simulink model "positive_negative_step_counters"  (R2019a)
settings: Solver=FixedStepDiscrete  StartTime=0.0  StopTime=50  FixedStep=1  RelTol=1e-3
settings Model: Creator=Suhas  LastModifiedBy=Suhas

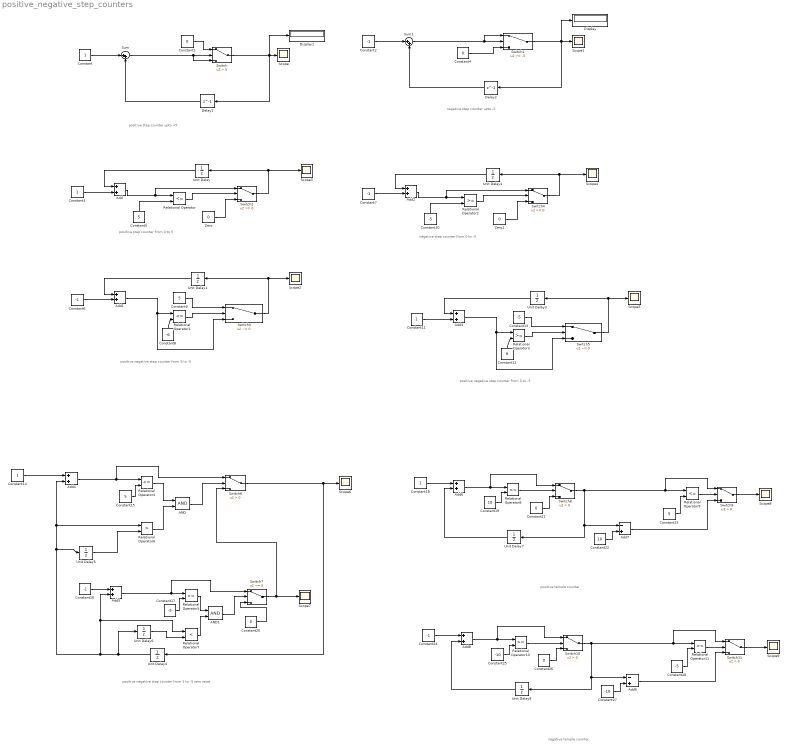
== system positive_negative_step_counters ==
  note: positive temple counter
  note: positive step counter from 0 to 5
  note: positive step counter upto +5
  note: negative step counter upto -5
  note: negative step counter from 0 to -5
  note: positive negative step counter from 5 to -5
  note: positive negative step counter from 5 to -5
  note: positive negative step counter from 5 to -5 zero reset
  note: negative temple counter
  AND : Logic  AllPortsSameDT=off  OutDataTypeStr=boolean
  AND1 : Logic  AllPortsSameDT=off  OutDataTypeStr=boolean
  Add{,1..6,8} (8 alike) : Sum
  Add7 : Sum  Inputs=-+
  Add9 : Sum  Inputs=-+
  Constant{,3,11,14,18} (5 alike) : Constant
  Constant{1,4,20..21,26} (5 alike) : Constant  Value=0
  Constant{10,13,17,28} (4 alike) : Constant  Value=-5
  Constant12 : Constant  Value=6
  Constant{5,9,15,23} (4 alike) : Constant  Value=5
  Constant{2,6..7,16,24} (5 alike) : Constant  Value=-1
  Constant19 : Constant  Value=10
  Constant22 : Constant  Value=10
  Constant25 : Constant  Value=-10
  Constant27 : Constant  Value=-10
  Constant8 : Constant  Value=-6
  Delay1 : Delay  DelayLength=1  InitialCondition=-1
  Delay2 : Delay  DelayLength=1  InitialCondition=1
  Display : Display
  Display1 : Display
  Relational Operator{,1,4,8..9} (5 alike) : RelationalOperator  Operator=<=  OutDataTypeStr=boolean  RndMeth=Simplest
  Relational Operator{2..3,5,10..11} (5 alike) : RelationalOperator  OutDataTypeStr=boolean  RndMeth=Simplest
  Relational Operator6 : RelationalOperator  Operator=>  OutDataTypeStr=boolean  RndMeth=Simplest
  Relational Operator7 : RelationalOperator  Operator=<  OutDataTypeStr=boolean  RndMeth=Simplest
  Scope{,1..9} (10 alike) : Scope
  Sum : Sum  Inputs=|++
  Sum1 : Sum  Inputs=|++
  Switch : Switch  Criteria=u2 > Threshold  Threshold=5
  Switch1 : Switch  Threshold=-5
  Switch{6,8..11} (5 alike) : Switch  Criteria=u2 > Threshold
  Switch2 : Switch
  Switch3 : Switch  Criteria=u2 ~= 0
  Switch4 : Switch
  Switch5 : Switch  Criteria=u2 ~= 0
  Switch7 : Switch  Criteria=u2 ~= 0
  Unit Delay{,3..4,7} (4 alike) : UnitDelay  InitialCondition=-1  SampleTime=-1  HasFrameUpgradeWarning=on
  Unit Delay1 : UnitDelay  InitialCondition=1  SampleTime=-1  HasFrameUpgradeWarning=on
  Unit Delay2 : UnitDelay  InitialCondition=1  SampleTime=-1  HasFrameUpgradeWarning=on
  Unit Delay5 : UnitDelay  InitialCondition=-2  SampleTime=-1  HasFrameUpgradeWarning=on
  Unit Delay6 : UnitDelay  SampleTime=-1  HasFrameUpgradeWarning=on
  Unit Delay8 : UnitDelay  InitialCondition=1  SampleTime=-1  HasFrameUpgradeWarning=on
  Zero : Constant  Value=0  OutDataTypeStr=Inherit: Inherit via back propagation
  Zero1 : Constant  Value=0  OutDataTypeStr=Inherit: Inherit via back propagation
  wires:
  Constant/1 -> Sum/1
  Sum/1 -> Switch/3, Switch/2
  Constant1/1 -> Switch/1
  Switch/1 -> Delay1/1, Display1/1, Scope/1
  Delay1/1 -> Sum/2
  Sum1/1 -> Switch1/1, Switch1/2
  Delay2/1 -> Sum1/2
  Constant2/1 -> Sum1/1
  Switch1/1 -> Display/1, Scope1/1, Delay2/1
  Constant4/1 -> Switch1/3
  Add/1 -> Switch2/1, Relational Operator/1
  Unit Delay/1 -> Add/1
  Constant3/1 -> Add/2
  Switch2/1 -> Scope3/1, Unit Delay/1
  Relational Operator/1 -> Switch2/2
  Constant5/1 -> Relational Operator/2
  Switch3/1 -> Scope2/1, Unit Delay1/1
  Constant6/1 -> Add1/2
  Add1/1 -> Relational Operator1/1, Switch3/3
  Constant8/1 -> Relational Operator1/2
  Unit Delay1/1 -> Add1/1
  Relational Operator1/1 -> Switch3/2
  Constant9/1 -> Switch3/1
  Zero/1 -> Switch2/3
  Zero1/1 -> Switch4/3
  Constant7/1 -> Add2/2
  Switch4/1 -> Scope4/1, Unit Delay2/1
  Constant10/1 -> Relational Operator2/2
  Relational Operator2/1 -> Switch4/2
  Add2/1 -> Switch4/1, Relational Operator2/1
  Unit Delay2/1 -> Add2/1
  Relational Operator3/1 -> Switch5/2
  Constant13/1 -> Switch5/1
  Unit Delay3/1 -> Add3/1
  Constant12/1 -> Relational Operator3/2
  Add3/1 -> Relational Operator3/1, Switch5/3
  Constant11/1 -> Add3/2
  Switch5/1 -> Scope5/1, Unit Delay3/1
  Unit Delay5/1 -> Relational Operator6/2
  Constant16/1 -> Add5/1
  Add5/1 -> Switch7/1, Relational Operator5/1
  Constant20/1 -> Switch7/3
  Switch7/1 -> Switch6/3, Scope7/1
  Unit Delay4/1 -> Unit Delay6/1, Relational Operator7/1, Add5/2, Add4/2, Relational Operator6/1, Unit Delay5/1
  Unit Delay6/1 -> Relational Operator7/2
  AND/1 -> Switch6/2
  Relational Operator4/1 -> AND/1
  AND1/1 -> Switch7/2
  Constant17/1 -> Relational Operator5/2
  Relational Operator6/1 -> AND/2
  Add4/1 -> Switch6/1, Relational Operator4/1
  Relational Operator7/1 -> AND1/2
  Relational Operator5/1 -> AND1/1
  Switch6/1 -> Scope6/1, Unit Delay4/1
  Constant14/1 -> Add4/1
  Constant15/1 -> Relational Operator4/2
  Constant18/1 -> Add6/1
  Add6/1 -> Switch8/1, Relational Operator8/1
  Constant19/1 -> Relational Operator8/2
  Relational Operator8/1 -> Switch8/2
  Constant21/1 -> Switch8/3
  Unit Delay7/1 -> Add6/2
  Constant22/1 -> Add7/2
  Constant23/1 -> Relational Operator9/2
  Switch8/1 -> Switch9/1, Relational Operator9/1, Unit Delay7/1, Add7/1
  Relational Operator9/1 -> Switch9/2
  Add7/1 -> Switch9/3
  Switch9/1 -> Scope8/1
  Constant26/1 -> Switch10/3
  Relational Operator10/1 -> Switch10/2
  Add9/1 -> Switch11/3
  Switch10/1 -> Switch11/1, Relational Operator11/1, Unit Delay8/1, Add9/1
  Switch11/1 -> Scope9/1
  Relational Operator11/1 -> Switch11/2
  Constant24/1 -> Add8/1
  Constant28/1 -> Relational Operator11/2
  Constant25/1 -> Relational Operator10/2
  Unit Delay8/1 -> Add8/2
  Add8/1 -> Switch10/1, Relational Operator10/1
  Constant27/1 -> Add9/2
